simulink model "modeloSimulink"  (R2018b)
settings: Solver=ode4  StartTime=0.0  StopTime=100  FixedStep=0.04  RelTol=1e-3
undefined symbols (not defined in the file): Angular, Linear
libraries: simulink x6, robotlib x4, fuzblock x1, Controllers x1
settings Model: Creator=root  LastModifiedBy=root

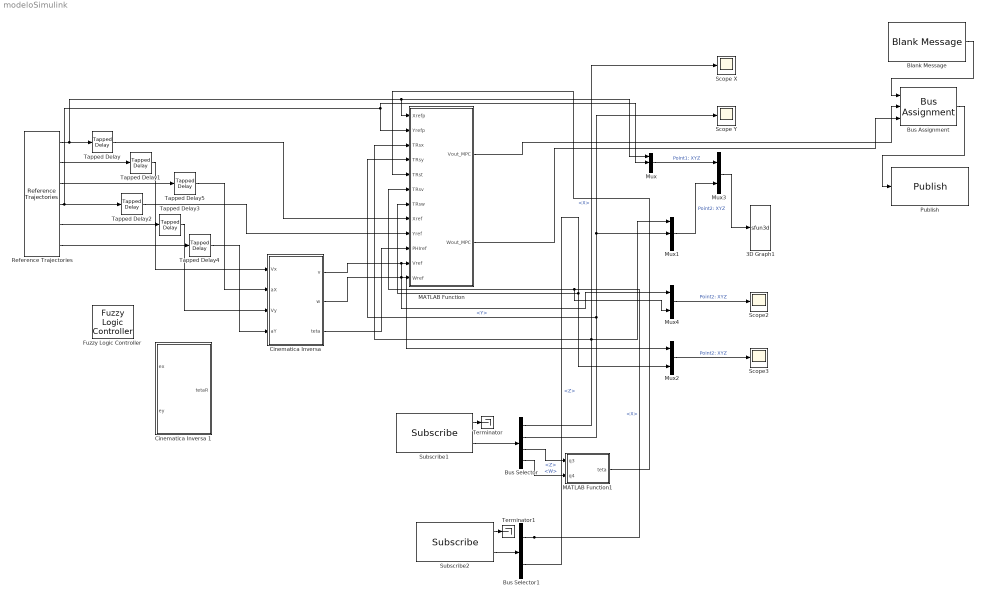
== system modeloSimulink ==
  3D Graph1 : S-Function  LoadFcn=if exist('sfun3d','file'), sfun3d([],[],[],'LoadBlock'); end  FunctionName=sfun3d  Parameters=ax,T,np,cp,gd,ls,mk,mx,hd,tb  SFunctionDeploymentMode=off  EnableBusSupport=off  mask(3D Graph){np=2, ax=[-4 4 -4 4 -3 3], mx=1e4, T=0.04, cp=[0 0 1], gd=on, hd=off, tb=off, ls=-, mk=none}
      mask prompts: np "Number of moving points (lines)"; ax "Range: [xmin xmax  ymin ymax zmin zmax]"; mx "Max number of points in each line"; T "Sampling Time"; cp "Camera position (use [0 0 1] for 2D XY view)"; gd "Grid (on|off)"; hd "HeadMarkers (on|off)"; tb "Toolbar (on|off)"; ls "LineStyle"; mk "LineMarker"
      mask help:
      | This block plots the position of several points in the XYZ space. The input contains the coordinates of all the points (x1,y1,z1,x2,y2,z2,...).
      | The number of moving points (lines), the XYZ ranges, sampling time, camera position, and grid (among other things) can be set as mask parameters.
      settings: CopyFcn=if exist('sfun3d','file'), sfun3d([],[],[],'CopyBlock'); end  DeleteFcn=if exist('sfun3d','file'), sfun3d([],[],[],'DeleteBlock'); end  NameChangeFcn=if exist('sfun3d','file'), sfun3d([],[],[],'NameChange'); end
      mask Help:
      | This block plots the position of several points in the XYZ space. The input contains the coordinates of all the points (x1,y1,z1,x2,y2,z2,...).
      | The number of moving points (lines), the XYZ ranges, sampling time, camera position, and grid (among other things) can be set as mask parameters.
      mask TypeOptions ls: - | -- | : | -. | none
      mask TypeOptions mk: none | . | + | o | * | x | square | diamond | v | ^ | > | < | pentagram | hexagram
      mask Display: plot([.05 .95 .95 .05 .05],[.45 .45 .95 .95 .45], 0.5+cos(0:0.1:2*pi)*0.3,0.7+sin(0:0.1:2*pi)*0.2)
  Blank Message : robotlib/Blank Message  messageClass=Message  entityType=geometry_msgs/Twist  messageType=geometry_msgs/Twist  SampleTime=inf
      settings: SourceProductBaseCode=RO
  Bus Assignment : BusAssignment  AssignedSignals=Linear.X,Angular.Z
  Bus Selector : BusSelector  OutputSignals=Pose.Pose.Position.X,Pose.Pose.Position.Y,Pose.Pose.Orientation.Z,Pose.Pose.Orientation.W
  Bus Selector1 : BusSelector  OutputSignals=Linear.X,Angular.Z
  "Cinematica Inversa " : MATLAB Function  TreatAsAtomicUnit=on
  Cinematica Inversa 1 : MATLAB Function  TreatAsAtomicUnit=on
  Fuzzy Logic Controller : fuzblock/Fuzzy Logic  Controller  FIS='fuzzy_rules.fis'  OutputSampleNumber=101  DataType=double  FuzzifiedInputs=off  RuleFiringStrengths=off  RuleOutputs=off  AggregatedOutputs=off  SimulateUsing=Interpreted execution  OutOfRangeInputValueMessage=warning  NoRuleFiredMessage=warning  EmptyOutputFuzzySetMessage=warning
  MATLAB Function : MATLAB Function  TreatAsAtomicUnit=on
  MATLAB Function1 : MATLAB Function  TreatAsAtomicUnit=on
  Mux : Mux  Inputs=3
  Mux1 : Mux  Inputs=3
  Mux2 : Mux  Inputs=2
  Mux3 : Mux  Inputs=2
  Mux4 : Mux  Inputs=2
  Publish : robotlib/Publish  topicSource=Select from ROS network  topic=/mobile_base/commands/velocity  messageType=geometry_msgs/Twist  messageQueueLength=1
      settings: SourceProductBaseCode=RO
  Reference Trajectories : Controllers/Reference Trajectories  trajectory_type=1  wf=0.10  raio_ref_1=1  delta_raio=0  t_delta_raio=60  xd=[1, -1.5]
  Scope X : Scope
  Scope Y : Scope
  Scope2 : Scope
  Scope3 : Scope
  Subscribe1 : robotlib/Subscribe  topicSource=Select from ROS network  topic=/odom  messageType=nav_msgs/Odometry  sampleTime=-1  messageQueueLength=1
      settings: SourceProductBaseCode=RO
  Subscribe2 : robotlib/Subscribe  topicSource=Select from ROS network  topic=/mobile_base/commands/velocity  messageType=geometry_msgs/Twist  sampleTime=-1  messageQueueLength=1
      settings: SourceProductBaseCode=RO
  Tapped Delay{,1..5} (6 alike) : simulink/Discrete/Tapped Delay  vinit=0.0  samptime=-1  NumDelays=1  DelayOrder=Oldest  includeCurrent=off
  Terminator : Terminator
  Terminator1 : Terminator
  wires:
  Mux1/1 -> Mux3/2  "Point2: XYZ"
  Mux/1 -> Mux3/1  "Point1: XYZ"
  Reference Trajectories/1 -> Tapped Delay/1, MATLAB Function/1(Xrefp), Mux/1
  Reference Trajectories/4 -> Tapped Delay2/1, MATLAB Function/2(Yrefp), Mux/2
  Reference Trajectories/2 -> Tapped Delay1/1
  Reference Trajectories/5 -> Tapped Delay3/1
  Reference Trajectories/6 -> Tapped Delay4/1
  Reference Trajectories/3 -> Tapped Delay5/1
  Tapped Delay/1 -> MATLAB Function/8(Xref)
  Tapped Delay2/1 -> MATLAB Function/9(Yref)
  "Cinematica Inversa "/1(v) -> Mux4/1, MATLAB Function/11(Vref)
  "Cinematica Inversa "/3(teta) -> MATLAB Function/10(PHIref)
  "Cinematica Inversa "/2(w) -> Mux2/1, MATLAB Function/12(Wref)
  Tapped Delay4/1 -> "Cinematica Inversa "/4(aY)
  Tapped Delay3/1 -> "Cinematica Inversa "/3(Vy)
  Tapped Delay5/1 -> "Cinematica Inversa "/2(aX)
  Tapped Delay1/1 -> "Cinematica Inversa "/1(Vx)
  Mux3/1 -> 3D Graph1/1
  MATLAB Function1/1(teta) -> MATLAB Function/5(TRst)
  MATLAB Function/1(Vout_MPC) -> Bus Assignment/2
  MATLAB Function/2(Wout_MPC) -> Bus Assignment/3
  Mux4/1 -> Scope2/1  "Point2: XYZ"
  Mux2/1 -> Scope3/1  "Point2: XYZ"
  Subscribe1/2 -> Bus Selector/1
  Bus Selector1/2 -> Mux2/2, MATLAB Function/7(TRsw)  "<Z>"
  Bus Selector1/1 -> Mux4/2, MATLAB Function/6(TRsv)  "<X>"
  Subscribe2/2 -> Bus Selector1/1
  Bus Assignment/1 -> Publish/1
  Subscribe2/1 -> Terminator1/1
  Bus Selector/2 -> Scope Y/1, Mux1/2, MATLAB Function/4(TRsy)  "<Y>"
  Bus Selector/4 -> MATLAB Function1/2(q4)  "<W>"
  Subscribe1/1 -> Terminator/1
  Blank Message/1 -> Bus Assignment/1
  Bus Selector/3 -> MATLAB Function1/1(q3)  "<Z>"
  Bus Selector/1 -> Scope X/1, MATLAB Function/3(TRsx), Mux1/1  "<X>"

== matlab function modeloSimulink/MATLAB Function1 ==
  data: q3 input; teta output; q4 input
function teta = fcn2(q3, q4)

    teta = 2*atan2(q3, q4);

end

== matlab function modeloSimulink/Cinematica Inversa 1 ==
  data: ex input; tetaR output; ey input
function tetaR  = fnc(ex, ey)
    tetaR = atan2(ex,ey);
end

== matlab function modeloSimulink/MATLAB Function ==
  data: Xrefp input; Vout_MPC output; Yrefp input; TRsx input; TRsy input; TRst input; TRsv input; TRsw input; Xref input; Yref input; PHIref input; Vref input; Wref input; Wout_MPC output
function [Vout_MPC, Wout_MPC] = MPC(Xrefp, Yrefp, TRsx, TRsy, TRst, TRsv, TRsw,Xref, Yref, PHIref, Vref, Wref)
    % Parâmetros do controlador
    Vmax = 0.4;
    d = 0.23;
    N1 = 1;
    N2 = 10; %Horizonte de predição
    Nu = 2;  %Horizonte de controle
    L1 = 10;    %1
    L2 = 2500;  %2.5
    L3 = 400;    %1
    eta = 0.1;
    Imax = 15;
    I = 0;
    Delta = 0.1;
    
    % Parâmetros do Otimizador
    alpha = 0.015;
    
    % Vetores do Otimizador
    
    Jgrad      = zeros([4 1]);
    Jgrad_prev = zeros([4 1]);
    Jsteps     = zeros([8 1]);
    % Definição das variáveis de controle
    
    Ubest = zeros([2 2]);
    Uref  = zeros([2 2]);
    Uaux  = zeros([2 2]);
    
    % Criação de um struct para guardar o valor da iteração anterior do
    % controlador
    SimRob = struct('x',0,'y',0,'teta',0,'v',0,'w',0);
    
    % Inicialização das variáveis de controle
    
    %Saida de controle desejada
    Uref = [Vref Vref; Wref Wref];
    
    % Cálculo da trajetoria de referencia
    lTi = 0;
    
    [tPX,tPY,tPTeta] = calcRefTraj(lTi,TRsx,TRsy,TRst,Xref,Yref,PHIref,Vref,Wref,N2,Xrefp,Yrefp);
    
    % Atualiza o modelo do preditor
    SimRob.x = TRsx;
    SimRob.y = TRsy;
    SimRob.teta = TRst;
    SimRob.v = TRsv;
    SimRob.w = TRsw;
    
    % Loop de controle
    
    % Reliza a saturaçao da velocidade das rodas com base na velocidade
    % máxima
    Uref = scaleForSaturation(Uref,d,Nu,Vmax);
    
    Jatual = COST_FUNCTION(SimRob.x,SimRob.y,SimRob.teta,SimRob.v,SimRob.w,Uref,tPX,tPY,tPTeta,N1,N2,Nu,L1,L2,L3);
    Jbest = Jatual;    

   %Loop de otimização do Ubest que minimiza o Jbest
   while (I < Imax) && (Jatual > eta)
       Usteps = calcUsteps(Uref,Nu, Delta);
        for k = 0:1:Nu-1
            for j=1:1:4
                %Atribui velocidade para cada passo U
                for m = 0:1:Nu-1
                    if m == k
                        Uaux(1,m+1)= Usteps(1,(j+4*k));
                        Uaux(2,m+1)= Usteps(2,(j+4*k));
                    else
                        Uaux(1,m+1)=Uref(1,1);
                        Uaux(2,m+1)=Uref(2,1);
                    end 
                    
                end
                SimRob.x=TRsx;
                SimRob.y=TRsy;
                SimRob.teta=TRst;
                SimRob.v=TRsv;
                SimRob.w=TRsw;

                Uaux=scaleForSaturation(Uaux,d,Nu,Vmax);

                J = COST_FUNCTION(SimRob.x,SimRob.y,SimRob.teta,SimRob.v,SimRob.w,Uaux,tPX,tPY,tPTeta,N1,N2,Nu,L1,L2,L3);
                Jsteps(j+ 4*k,1) = J;
            
            end
        end
        
        % calculo do gradiente de J baseado no Jsteps
        for h=0:1:Nu-1
            Jgrad_prev(2*h+1,1) = Jgrad(2*h+1,1);
            Jgrad(2*h+1,1) = Jsteps(4*h+1,1)- Jsteps(4*h+2,1);
            Jgrad_prev(2*h+2,1) = Jgrad(2*h+2,1);
            Jgrad(2*h+2,1)=Jsteps(4*h+3,1)-Jsteps(4*h+4,1);
        end
    
        %Gradiente conjugado Algoritmo de Polak-Bibieri

        di=[0 0];
        x1=di;

        for z=0:1:Nu-1
            di(1)=Jgrad(2*z+1,1);
            di(2)=Jgrad(2*z+2,1);
            
            x1(1)=(Uref(1,z+1) - alpha*di(1));
            x1(2)=(Uref(2,z+1) - alpha*di(2));
            
            Jgrad_prev(2*z+1,1)=Jgrad(2*z+1,1);
            Jgrad(2*z+1,1)=Jsteps(4*z+1,1)-Jsteps(4*z+2,1);
            
            Jgrad_prev(2*z+2,1)=Jgrad(2*z+2,1);
            Jgrad(2*z+2,1)=Jsteps(4*z+3,1)-Jsteps(4*z+4,1);
            
            beta=0;
            
            if ((Jgrad(2*z+1,1)>=eta)||(Jgrad(2*z+2,1)>=eta))
                
                t1=(Jgrad(2*z+1,1)-Jgrad_prev(2*z+1,1));
                t2=(Jgrad(2*z+2,1)-Jgrad_prev(2*z+2,1));
                
                a1=(Jgrad(2*z+1,1)*t1);
                a2=(Jgrad(2*z+2,1)*t2);
               
                b1=(Jgrad_prev(2*z+1,1)*Jgrad_prev(2*z+1,1));
                b2=(Jgrad_prev(2*z+2,1)*Jgrad_prev(2*z+2,1));
                
                beta=((a1+a2)/(b1+b2));
            
            end
            
            Uref(1,z+1)=x1(1)+alpha*(-Jgrad(2*z+1,1)+beta*Jgrad_prev(2*z+1,1));

            Uref(2,z+1)=x1(2)+alpha*(-Jgrad(2*z+2,1)+beta*Jgrad_prev(2*z+2,1));
        end
        
        
        SimRob.x=TRsx;
        SimRob.y=TRsy;
        SimRob.teta=TRst;
        SimRob.v=TRsv;
        SimRob.w=TRsw;
        
        % ix SATURA A VELOCIDADE DAS RODAS QUE SERÃO USADAS NO PRÓXIMO LOOP
        % DE CONTROLE (while)
        
        Uref = scaleForSaturation(Uref,d,Nu,Vmax);
        
        Jatual = COST_FUNCTION(SimRob.x,SimRob.y,SimRob.teta,SimRob.v,SimRob.w,Uref,tPX,tPY,tPTeta,N1,N2,Nu,L1,L2,L3);
        
        if Jatual < Jbest
            Jbest = Jatual;
            Ubest = Uref;
        end
        I=I+1;
    end %END_WHILE      
    Vout_MPC = Ubest(1,1);
    Wout_MPC = Ubest(2,1);

== matlab function modeloSimulink/Cinematica Inversa  ==
  data: Vx input; v output; aX input; Vy input; aY input; w output; teta output
function [v,w,teta] = fnc(Vx, aX, Vy, aY)
  
    teta = atan2(Vy,Vx);
    
    v = sqrt(Vx^2 + Vy^2);
    
    w = (Vx*aY - Vy*aX)/(Vx^2 + Vy^2);

end
